simulink model "HXpump_justplant"  (R2013a)
settings: Solver=FixedStepDiscrete  StartTime=0.0  StopTime=Tfinal  FixedStep=Ts  RelTol=1e-3
values from neighbouring files (symbols this model uses):
  A = wallpar(4)    [EKFdynamics.m]    (also in heatexchanger.m; heatexchangerpump.m; hxpumpcode.m = params.A; hxpumpcodesanity.m = 292.2)
  cc = coldpar(3)    [EKFdynamics.m]    (also in heatexchanger.m; heatexchangerpump.m; hxpumpcode.m = params.cc; hxpumpcodesanity.m = 1901)
  ch = hotpar(3)    [EKFdynamics.m]    (also in heatexchanger.m; heatexchangerpump.m; hxpumpcode.m = params.ch; hxpumpcodesanity.m = 2414)
  cw = wallpar(3)    [EKFdynamics.m]    (also in heatexchanger.m; heatexchangerpump.m; hxpumpcode.m = params.cw; hxpumpcodesanity.m = 578)
  hc = coldpar(4)    [EKFdynamics.m]    (also in heatexchanger.m; heatexchangerpump.m; hxpumpcode.m = params.hc; hxpumpcodesanity.m = 24500)
  hh = hotpar(5)    [EKFdynamics.m]    (also in heatexchanger.m; heatexchangerpump.m; hxpumpcode.m = params.hh; hxpumpcodesanity.m = 23800)
  ki = 1.2    [HeatExchanger_ps.m]    (also in hxpumpcode.m = 1; hxpumpcodesanity.m; noErrornoDelay.mat = 1)
  kp = 4.995    [HeatExchanger_ps.m]    (also in hxpumpcode.m = 4; hxpumpcodesanity.m; noErrornoDelay.mat = 4)
  mdoth = hotpar(4)    [EKFdynamics.m]    (also in heatexchanger.m; heatexchangerpump.m; hxpumpcode.m = params.mdoth; hxpumpcodesanity.m = 350)
  Pref = params.Pref    [hxpumpcode.m]    (also in hxpumpcodesanity.m = 37.8; noErrornoDelay.mat = 37.8)
  rhoc = coldpar(1)    [EKFdynamics.m]    (also in heatexchanger.m; heatexchangerpump.m; hxpumpcode.m = params.rhoc; hxpumpcodesanity.m = 2020)
  rhoh = hotpar(1)    [EKFdynamics.m]    (also in heatexchanger.m; heatexchangerpump.m; hxpumpcode.m = params.rhoh; hxpumpcodesanity.m = 1940)
  rhow = wallpar(1)    [EKFdynamics.m]    (also in heatexchanger.m; heatexchangerpump.m; hxpumpcode.m = params.rhow; hxpumpcodesanity.m = 8860)
  Tci = input(2)    [EKFdynamics.m]    (also in heatexchanger.m; heatexchangerpump.m; hxpumpcode.m = params.Tci; hxpumpcodesanity.m = 550)
  Thi = hotpar(6)    [EKFdynamics.m]    (also in heatexchanger.m; heatexchangerpump.m; hxpumpcode.m = params.Thi; hxpumpcodesanity.m = 700)
  Ts = delta_t    (= 0.1)    [HeatExchanger_ps.m]    (also in hxpumpcode.m = params.Ts; hxpumpcodesanity.m; noErrornoDelay.mat)
  Vc = coldpar(2)    [EKFdynamics.m]    (also in heatexchanger.m; heatexchangerpump.m; hxpumpcode.m = params.Vc; hxpumpcodesanity.m = 1.5127)
  Vh = hotpar(2)    [EKFdynamics.m]    (also in heatexchanger.m; heatexchangerpump.m; hxpumpcode.m = params.Vh; hxpumpcodesanity.m = 1.1508)
  Vw = wallpar(2)    [EKFdynamics.m]    (also in heatexchanger.m; heatexchangerpump.m; hxpumpcode.m = params.Vw; hxpumpcodesanity.m = 0.4675)
  wp = pumppar(1)    [EKFdynamics.m]    (also in heatexchangerpump.m; hxpumpcode.m = params.wp; hxpumpcodesanity.m = 0.1; noErrornoDelay.mat = 0.1)
  x0 = tempx0'    [hxpumpcode.m]    (also in hxpumpcodesanity.m = [650.29 638.4 644.3 mdoth Thi 250]; noErrornoDelay.mat = [655.2 644.46 649.75 350 700 210.8])
settings Model: Creator=LabUser  LastModifiedBy=LabUser
settings DataIOCC: LimitDataPoints=off

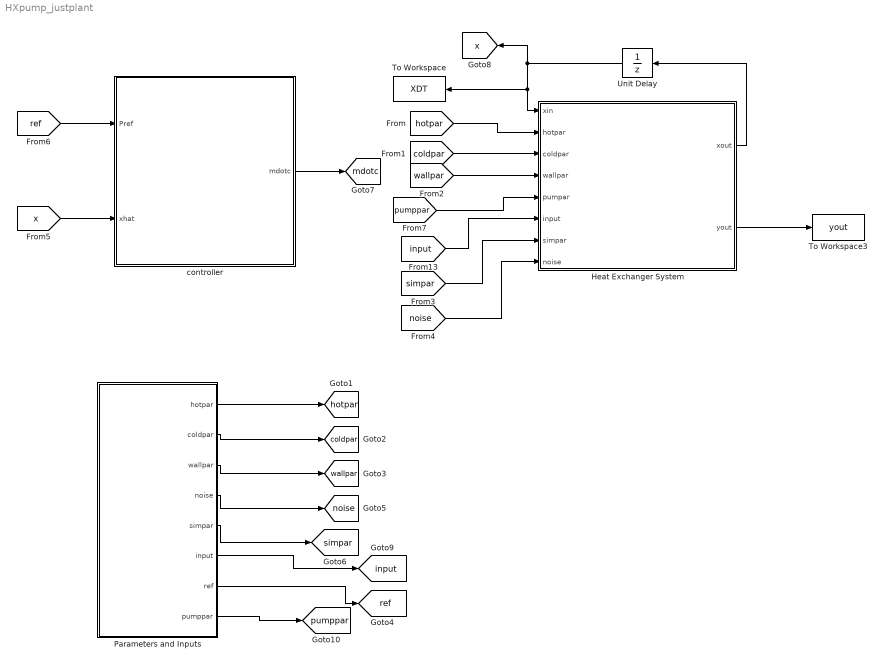
== system HXpump_justplant ==
  Heat Exchanger System : MATLAB Function  TreatAsAtomicUnit=on
  Parameters and Inputs : Subsystem
  To Workspace : ToWorkspace  VariableName=XDT  SampleTime=-1
  To Workspace3 : ToWorkspace  VariableName=yout  SampleTime=-1
  Unit Delay : UnitDelay  InitialCondition=x0([1 2 3 6])  SampleTime=-1
  controller : Subsystem
  tag scope: coldpar=global, hotpar=global, input=global, mdotc=global, noise=global, pumppar=global, ref=global, simpar=global, wallpar=global, x=global
  wires:
  Unit Delay/1 -> [x], To Workspace/1, Heat Exchanger System/1(xin)
  Heat Exchanger System/1(xout) -> Unit Delay/1
  [hotpar] -> Heat Exchanger System/2(hotpar)
  [coldpar] -> Heat Exchanger System/3(coldpar)
  [wallpar] -> Heat Exchanger System/4(wallpar)
  [simpar] -> Heat Exchanger System/7(simpar)
  [noise] -> Heat Exchanger System/8(noise)
  Parameters and Inputs/1(hotpar) -> [hotpar]
  Parameters and Inputs/2(coldpar) -> [coldpar]
  Parameters and Inputs/3(wallpar) -> [wallpar]
  Parameters and Inputs/4(noise) -> [noise]
  Parameters and Inputs/5(simpar) -> [simpar]
  Heat Exchanger System/2(yout) -> To Workspace3/1
  Parameters and Inputs/6(input) -> [input]
  [input] -> Heat Exchanger System/6(input)
  Parameters and Inputs/7(ref) -> [ref]
  [ref] -> controller/1(Pref)
  [x] -> controller/2(xhat)
  controller/1(mdotc) -> [mdotc]
  Parameters and Inputs/8(pumppar) -> [pumppar]
  [pumppar] -> Heat Exchanger System/5(pumpar)

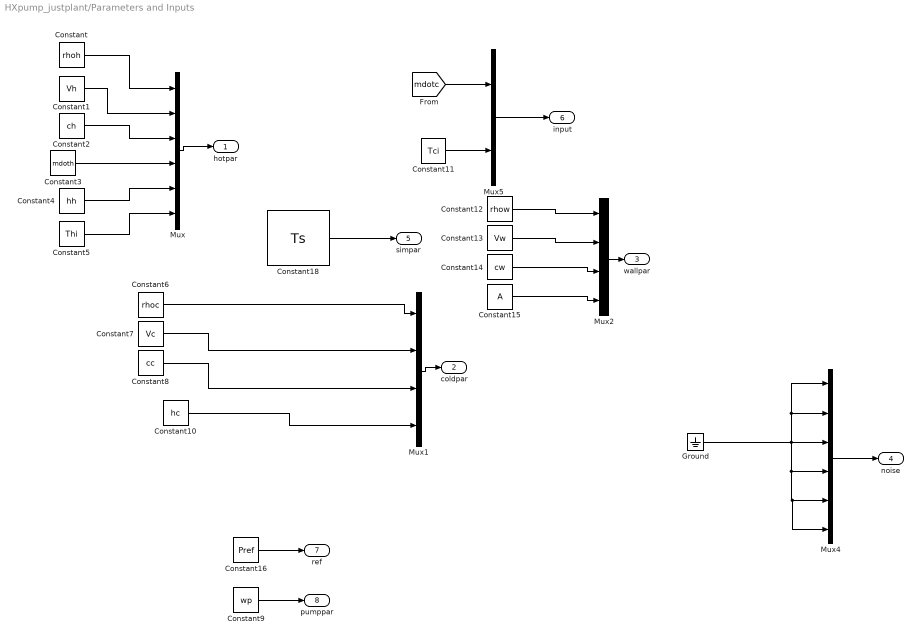
== system HXpump_justplant/Parameters and Inputs ==
  Constant : Constant  Value=rhoh  SampleTime=Ts
  Constant1 : Constant  Value=Vh  SampleTime=Ts
  Constant10 : Constant  Value=hc  SampleTime=Ts
  Constant11 : Constant  Value=Tci  SampleTime=Ts
  Constant12 : Constant  Value=rhow  SampleTime=Ts
  Constant13 : Constant  Value=Vw  SampleTime=Ts
  Constant14 : Constant  Value=cw  SampleTime=Ts
  Constant15 : Constant  Value=A  SampleTime=Ts
  Constant16 : Constant  Value=Pref  SampleTime=Ts
  Constant18 : Constant  Value=Ts  SampleTime=Ts
  Constant2 : Constant  Value=ch  SampleTime=Ts
  Constant3 : Constant  Value=mdoth  SampleTime=Ts
  Constant4 : Constant  Value=hh  SampleTime=Ts
  Constant5 : Constant  Value=Thi  SampleTime=Ts
  Constant6 : Constant  Value=rhoc  SampleTime=Ts
  Constant7 : Constant  Value=Vc  SampleTime=Ts
  Constant8 : Constant  Value=cc  SampleTime=Ts
  Constant9 : Constant  Value=wp  SampleTime=Ts
  Ground : Ground
  Mux : Mux  Inputs=6
  Mux1 : Mux
  Mux2 : Mux
  Mux4 : Mux  Inputs=6
  Mux5 : Mux  Inputs=2
  hotpar : Outport
  coldpar : Outport  Port=2
  wallpar : Outport  Port=3
  noise : Outport  Port=4
  simpar : Outport  Port=5
  input : Outport  Port=6
  ref : Outport  Port=7
  pumppar : Outport  Port=8
  wires:
  Constant1/1 -> Mux/2
  Constant/1 -> Mux/1
  Mux/1 -> hotpar/1
  Constant2/1 -> Mux/3
  Constant6/1 -> Mux1/1
  Mux1/1 -> coldpar/1
  Constant8/1 -> Mux1/3
  Constant7/1 -> Mux1/2
  Mux2/1 -> wallpar/1
  Constant10/1 -> Mux1/4
  Constant12/1 -> Mux2/1
  Constant13/1 -> Mux2/2
  Constant14/1 -> Mux2/3
  Constant15/1 -> Mux2/4
  Mux4/1 -> noise/1
  Constant18/1 -> simpar/1
  Constant4/1 -> Mux/5
  Mux5/1 -> input/1
  [mdotc] -> Mux5/1
  Constant11/1 -> Mux5/2
  Constant3/1 -> Mux/4
  Constant5/1 -> Mux/6
  Ground/1 -> Mux4/1, Mux4/2, Mux4/4, Mux4/5, Mux4/6, Mux4/3
  Constant16/1 -> ref/1
  Constant9/1 -> pumppar/1

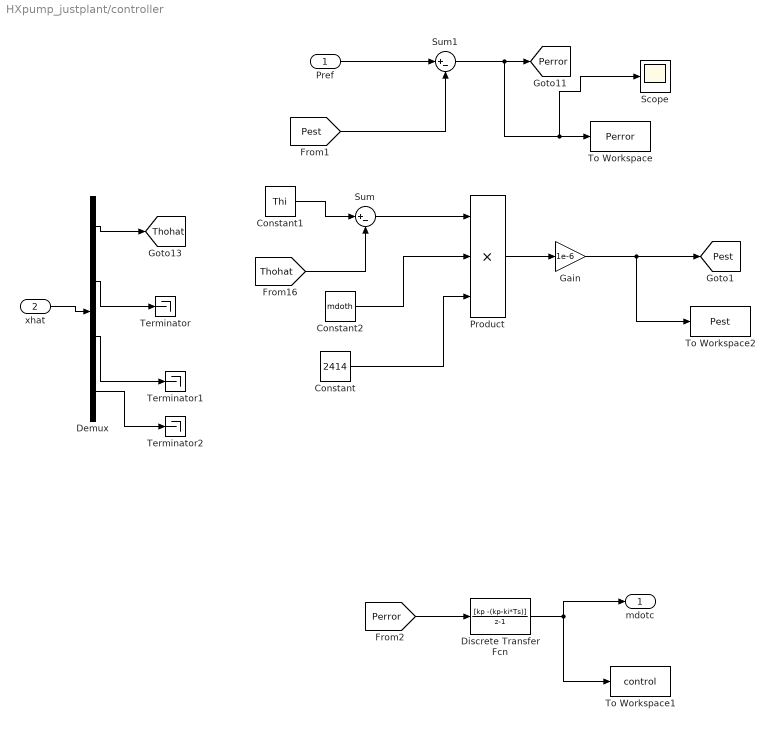
== system HXpump_justplant/controller ==
  Pref : Inport
  xhat : Inport  Port=2
  Constant : Constant  Value=2414  SampleTime=Ts
  Constant1 : Constant  Value=Thi  SampleTime=Ts
  Constant2 : Constant  Value=mdoth  SampleTime=Ts
  Demux : Demux
  Discrete Transfer Fcn : DiscreteTransferFcn  Numerator=[kp -(kp-ki*Ts)]  Denominator=[1 -1]  InitialStates=20  SampleTime=Ts
  Gain : Gain  Gain=1e-6
  Product : Product  Inputs=3
  Scope : Scope
  Sum : Sum  Inputs=|+-
  Sum1 : Sum  Inputs=|+-
  Terminator : Terminator
  Terminator1 : Terminator
  Terminator2 : Terminator
  To Workspace : ToWorkspace  VariableName=Perror  SampleTime=-1
  To Workspace1 : ToWorkspace  VariableName=control  SampleTime=-1
  To Workspace2 : ToWorkspace  VariableName=Pest  SampleTime=-1
  mdotc : Outport
  tag scope: Perror=global, Pest=global, Thohat=global
  wires:
  Demux/3 -> Terminator1/1
  [Thohat] -> Sum/2
  Constant2/1 -> Product/2
  Sum/1 -> Product/1
  Constant/1 -> Product/3
  Demux/1 -> [Thohat]
  Constant1/1 -> Sum/1
  xhat/1 -> Demux/1
  Demux/2 -> Terminator/1
  Product/1 -> Gain/1
  Pref/1 -> Sum1/1
  Gain/1 -> To Workspace2/1, [Pest]
  [Pest] -> Sum1/2
  Sum1/1 -> To Workspace/1, Scope/1, [Perror]
  Discrete Transfer Fcn/1 -> mdotc/1, To Workspace1/1
  [Perror] -> Discrete Transfer Fcn/1
  Demux/4 -> Terminator2/1

== matlab function HXpump_justplant/Heat Exchanger System ==
  data: xin input; xout output; hotpar input; coldpar input; wallpar input; pumpar input; input input; simpar input; noise input; yout output
function [xout,yout] = fcn(xin,hotpar,coldpar,wallpar,pumpar,input,simpar,noise)
%#codegen

% simulation parameters
h = simpar(1);

% Sensor noise
v_thi = noise(4);
v_tho = noise(5);
v_mh  = noise(6);
v = [v_thi ; v_tho ; v_mh];

% hot-leg parameters
Thi   = hotpar(6);
mdoth = hotpar(4);

% fourth order Runga Kutta

c1 = 1/6;
c2 = 1/3;
c3 = 1/3;
c4 = 1/6;
a2 = 1/2;
a3 = 1/2;
a4 = 1;
b21 = 1/2;
b31 = 0;
b32 = 1/2;
b41 = 0;
b42 = 0;
b43 = 1;

%%%%% System dynamics

K1 = heatexchangerpump(xin,hotpar,coldpar,wallpar,pumpar,input,noise);
K2 = heatexchangerpump(xin+b21*K1*h,hotpar,coldpar,wallpar,pumpar,input,noise);
K3 = heatexchangerpump(xin+b31*K1*h+b32*K2*h,hotpar,coldpar,wallpar,pumpar,input,noise);
K4 = heatexchangerpump(xin+b41*K1*h+b42*K2*h+b43*K3*h,hotpar,coldpar,wallpar,pumpar,input,noise);
slope = c1*K1+c2*K2+c3*K3+c4*K4;

xout = xin + slope*h;
yout = [Thi; xin(1); mdoth] + eye(3)*v;
